simulink model "Dynamics"  (R2025b)
settings: Solver=ode45  StartTime=0.0  StopTime=5  RelTol=1e-6
settings Model: Creator=maiaelizabethgorham  LastModifiedBy=ryan

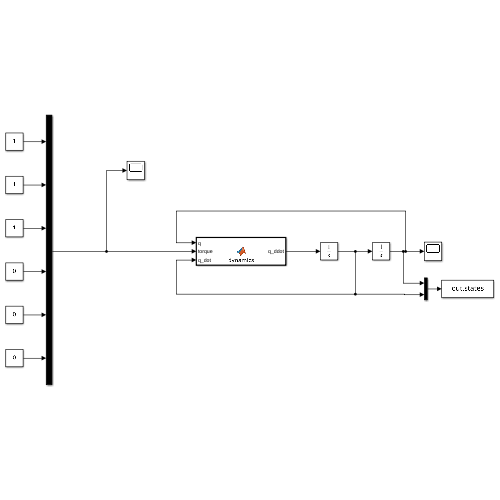
[thumbnail: Simulink's stored preview of the top-level diagram]
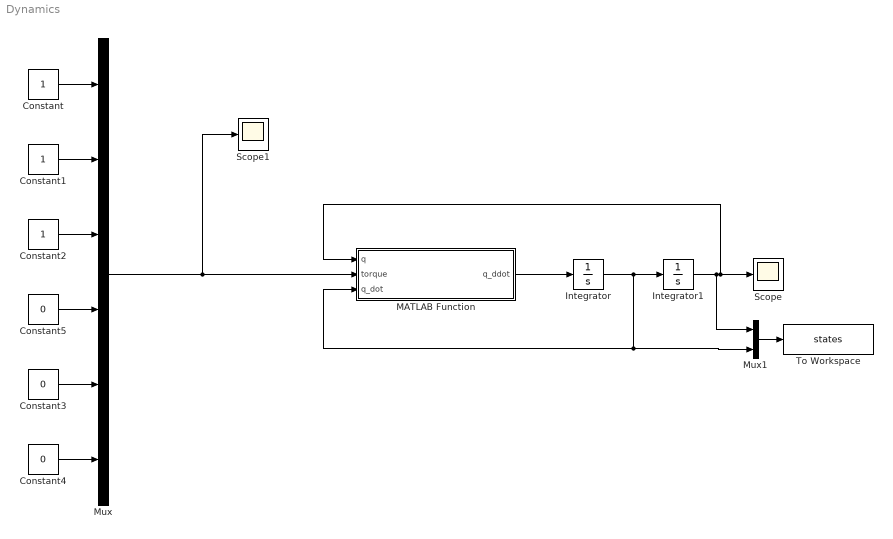
== system Dynamics ==
  Constant : Constant
  Constant1 : Constant
  Constant2 : Constant
  Constant3 : Constant  Value=0
  Constant4 : Constant  Value=0
  Constant5 : Constant  Value=0
  Integrator : Integrator  InitialCondition=[0;0;0;0;0;0]
  Integrator1 : Integrator  InitialCondition=[0;0;0;0;0;0]
  MATLAB Function : MATLAB Function  TreatAsAtomicUnit=on
  Mux : Mux  Inputs=6
  Mux1 : Mux  Inputs=2
  Scope : Scope
      settings: ActiveDisplayYMinimum=-1  ActiveDisplayYMaximum=1
  Scope1 : Scope
      settings: ActiveDisplayYMinimum=-1  ActiveDisplayYMaximum=1
  To Workspace : ToWorkspace  VariableName=states  SaveFormat=Timeseries  SampleTime=-1
  wires:
  Integrator/1 -> Mux1/2, MATLAB Function/3(q_dot), Integrator1/1
  MATLAB Function/1(q_ddot) -> Integrator/1
  Integrator1/1 -> Mux1/1, MATLAB Function/1(q), Scope/1
  Mux/1 -> Scope1/1, MATLAB Function/2(torque)
  Constant/1 -> Mux/1
  Constant3/1 -> Mux/5
  Constant4/1 -> Mux/6
  Constant1/1 -> Mux/2
  Constant2/1 -> Mux/3
  Constant5/1 -> Mux/4
  Mux1/1 -> To Workspace/1

== matlab function Dynamics/MATLAB Function ==
  settings: updateMethod=CONTINUOUS  sampleTime=0.01
  data: q input; torque input; q_dot input; q_ddot output
function q_ddot = dynamics(q, torque, q_dot)

d2r = pi/180;
r2d = 1/d2r;

I0 = 0.2873675;         %kg*m^2
I1 = 0.0037502;         %kg*m^2
I2 = 0.0034132;         %kg*m^2
I3 = 0.000056402588;    %kg*m^2

phi = 68.2840*d2r;      %rad
b0 = 0.2304;            %m

a1 = 0.1933;            %m
b1 = 0.1117;            %m
a2 = 0.1993;            %m
b2 = 0.1057;            %m
a3 = 0.0621;            %m
b3 = 0.0159;            %m

m0 = 16.9478;           %kg
m1 = 0.3434;            %kg
m2 = 0.3334;            %kg
m3 = 0.0111;            %kg

x0 = q(1);
y0 = q(2);
q0 = q(3);
q1 = q(4);
q2 = q(5);
q3 = q(6);

x0_dot = q_dot(1);
y0_dot = q_dot(2);
q0_dot = q_dot(3);
q1_dot = q_dot(4);
q2_dot = q_dot(5);
q3_dot = q_dot(6);

M = InertiaFunc3LINK(I0,I1,I2,I3,a1,a2,a3,b0,b1,b2,m0,m1,m2,m3,phi,q0,q1,q2,q3);

C = CoriolisFunc3LINK(a1,a2,a3,b0,b1,b2,m1,m2,m3,phi,q0,q1,q2,q3,q0_dot,q1_dot,q2_dot,q3_dot);

q_ddot = M\(torque - C*q_dot);

end
